simulink model "p9"  (R2020a)
settings: Solver=VariableStepAuto  StartTime=0.0  StopTime=10.0  RelTol=1e-3
undefined symbols (not defined in the file or in its folder): B, J, P
settings Model: Creator=007  LastModifiedBy=007

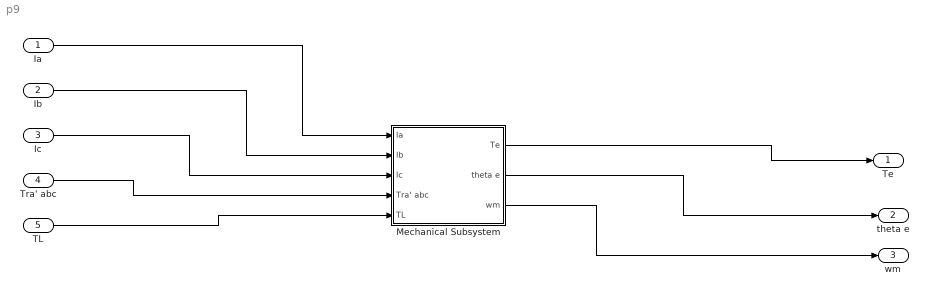
== system p9 ==
  Ia : Inport
  Ib : Inport  Port=2
  Ic : Inport  Port=3
  Tra' abc : Inport  Port=4
  TL : Inport  Port=5
  Mechanical Subsystem : Subsystem
  Te : Outport
  theta e : Outport  Port=2
  wm : Outport  Port=3
  wires:
  Ia/1 -> Mechanical Subsystem/1(Ia)
  Ib/1 -> Mechanical Subsystem/2(Ib)
  Ic/1 -> Mechanical Subsystem/3(Ic)
  Tra' abc/1 -> Mechanical Subsystem/4(Tra' abc)
  TL/1 -> Mechanical Subsystem/5(TL)
  Mechanical Subsystem/1(Te) -> Te/1
  Mechanical Subsystem/2(theta e) -> theta e/1
  Mechanical Subsystem/3(wm) -> wm/1

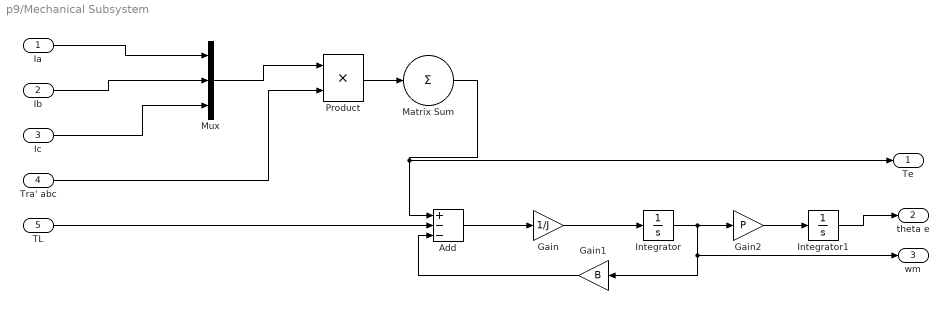
== system p9/Mechanical Subsystem ==
  Ia : Inport
  Ib : Inport  Port=2
  Ic : Inport  Port=3
  Tra' abc : Inport  Port=4
  TL : Inport  Port=5
  Add : Sum  Inputs=+--
  Gain : Gain  Gain=1/J
  Gain1 : Gain  Gain=B
  Gain2 : Gain  Gain=P
  Integrator : Integrator
  Integrator1 : Integrator
  Matrix Sum : Sum  Inputs=+
  Mux : Mux  Inputs=3
  Product : Product
  Te : Outport
  theta e : Outport  Port=2
  wm : Outport  Port=3
  wires:
  Ib/1 -> Mux/2
  Matrix Sum/1 -> Te/1, Add/1
  Ia/1 -> Mux/1
  Tra' abc/1 -> Product/2
  Integrator1/1 -> theta e/1
  Product/1 -> Matrix Sum/1
  Integrator/1 -> Gain2/1, wm/1, Gain1/1
  Gain1/1 -> Add/3
  Gain/1 -> Integrator/1
  TL/1 -> Add/2
  Gain2/1 -> Integrator1/1
  Mux/1 -> Product/1
  Add/1 -> Gain/1
  Ic/1 -> Mux/3
